simulink model "pid_sim"  (R2025b)
settings: Solver=ode3  StartTime=0.0  StopTime=Endtime  FixedStep=1  RelTol=1e-3
values from neighbouring files (symbols this model uses):
  d0 = 25.0    (= 25)    [Ex4_2.m]    (also in Ex4_2_1.m; pid_hw.m)
  K = 1.15    [Ex4_2.m]    (also in Ex4_2_1.m; pid_hw.m)
  kc = 0.6*T/(K*L)    (= 38.7826086957)    [Ex4_2.m]    (also in Ex4_2_1.m; pid_hw.m = P(i,1))
  L = 15    [Ex4_2.m]    (also in Ex4_2_1.m; pid_hw.m = 150)
  r = 50    [Ex4_2.m]    (also in Ex4_2_1.m; pid_hw.m)
  T = 1115    [Ex4_2.m]    (also in Ex4_2_1.m; pid_hw.m)
  Td = 0.5*L    (= 7.5)    [Ex4_2.m]    (also in Ex4_2_1.m; pid_hw.m = P(i,3))
  Ti = T    (= 1115)    [Ex4_2.m]    (also in Ex4_2_1.m; pid_hw.m = P(i,2))
  Tswitch = (i > 1)*1    [pid_hw.m]
settings Model: Creator=Shin
settings SolverCC: AlgebraicLoopSolver=TrustRegion
settings DataIOCC: LimitDataPoints=on  SaveFormat=Array  ReturnWorkspaceOutputs=off
settings OptimizationCC: BlockReduction=off  BooleanDataType=off  LifeSpan=inf
settings DebuggingCC: SaveWithParameterizedLinksMsg=none  UnderspecifiedInitializationDetection=Classic  MergeDetectMultiDrivingBlocksExec=none  SignalResolutionControl=TryResolveAllWithWarning  UnconnectedInputMsg=warning  UnconnectedOutputMsg=warning  UnconnectedLineMsg=warning  SFUnexpectedBacktrackingDiag=warning  SFNoUnconditionalDefaultTransitionDiag=warning  SFExecutionAtInitializationDiag=none  ArithmeticOperatorsInVariantConditions=warning
settings HardwareCC: ProdBitPerPointer=32.0  ProdBitPerSizeT=32.0  ProdBitPerPtrDiffT=32.0  ProdLargestAtomicFloat=None  ProdIntDivRoundTo=Undefined  ProdEndianess=Unspecified  ProdWordSize=32.0  ProdHWDeviceType=32-bit Generic  TargetUnknown=on
settings ModelReferenceCC: PropagateSignalLabelsOutOfModel=off
settings SFSimCC: SimUseLocalCustomCode=off  CustomCodeUndefinedFunction=UseInterfaceOnly
settings RTWCC: RTWUseLocalCustomCode=off  GPUComputeCapability=3.5
settings CodeAppCC: StateflowObjectComments=on
settings GRTTargetCC: TargetLangStandard=C89/C90 (ANSI)
settings ConfigComp: CovMetricSettings=dw  CovSaveCumulativeToWorkspaceVar=on  CovSaveSingleToWorkspaceVar=on  CovExternalEMLEnable=off  CovSFcnEnable=off

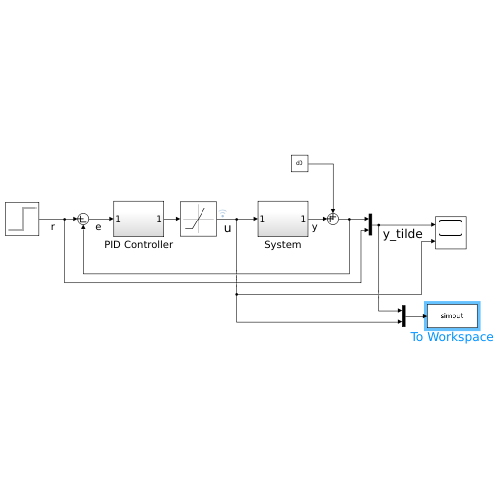
[thumbnail: Simulink's stored preview of the top-level diagram]
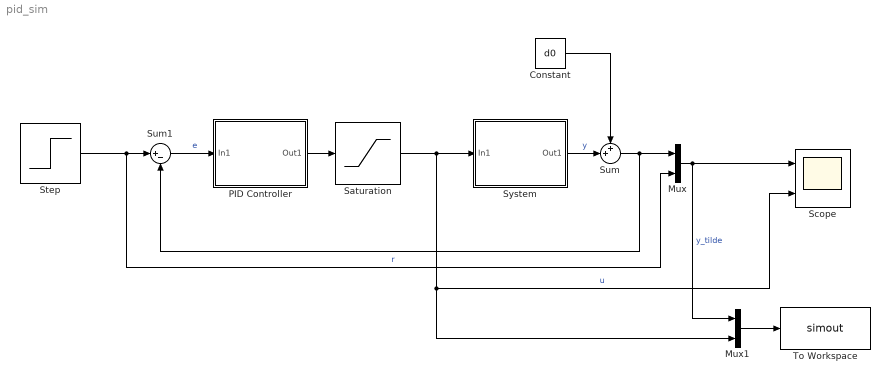
== system pid_sim ==
  Constant : Constant  Value=d0
  Mux : Mux  Inputs=2
  Mux1 : Mux  Inputs=2
  PID Controller : Subsystem
  Saturation : Saturate  UpperLimit=300  LowerLimit=0
  Scope : Scope  NumInputPorts=2
      settings: ActiveDisplayYMinimum=24.651923197379507  ActiveDisplayYMaximum=58.460292635310054  DataLoggingSaveFormat=Array
  Step : Step  After=r  SampleTime=0
  Sum : Sum  Inputs=++|
  Sum1 : Sum  Inputs=|+-
  System : Subsystem
  To Workspace : ToWorkspace  VariableName=simout  SaveFormat=Timeseries  SampleTime=-1
  wires:
  System/1(Out1) -> Sum/2  "y"
  Step/1 -> Mux/2, Sum1/1  "r"
  Constant/1 -> Sum/1
  Sum/1 -> Mux/1, Sum1/2
  PID Controller/1(Out1) -> Saturation/1
  Sum1/1 -> PID Controller/1(In1)  "e"
  Mux/1 -> Mux1/1, Scope/1  "y_tilde"
  Saturation/1 -> System/1(In1), Mux1/2, Scope/2  "u"
  Mux1/1 -> To Workspace/1

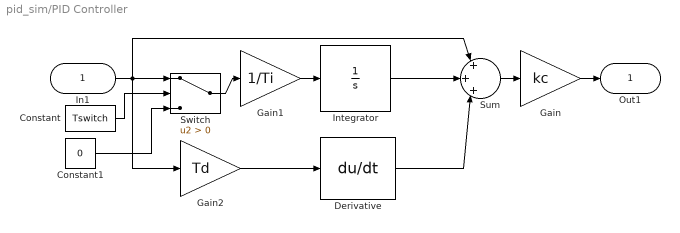
== system pid_sim/PID Controller ==
  In1 : Inport
  Constant : Constant  Value=Tswitch
  Constant1 : Constant  Value=0
  Derivative : Derivative
  Gain : Gain  Gain=kc
  Gain1 : Gain  Gain=1/Ti
  Gain2 : Gain  Gain=Td
  Integrator : Integrator
  Sum : Sum  Inputs=|+|+|+|
  Switch : Switch  Criteria=u2 > Threshold  SaturateOnIntegerOverflow=off  InputSameDT=off
  Out1 : Outport
  wires:
  In1/1 -> Switch/1, Sum/1, Gain2/1
  Sum/1 -> Gain/1
  Gain/1 -> Out1/1
  Gain1/1 -> Integrator/1
  Gain2/1 -> Derivative/1
  Integrator/1 -> Sum/2
  Derivative/1 -> Sum/3
  Switch/1 -> Gain1/1
  Constant/1 -> Switch/2
  Constant1/1 -> Switch/3

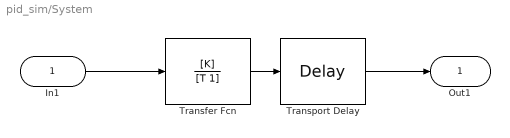
== system pid_sim/System ==
  In1 : Inport
  Transfer Fcn : TransferFcn  Numerator=[K]  Denominator=[T 1]
  Transport Delay : TransportDelay  DelayTime=L
  Out1 : Outport
  wires:
  Transport Delay/1 -> Out1/1
  Transfer Fcn/1 -> Transport Delay/1
  In1/1 -> Transfer Fcn/1
